simulink model "NPW_Model"  (R2025a)
settings: Solver=VariableStepAuto  StartTime=0.0  StopTime=150.0  RelTol=1e-3
undefined symbols (not defined in the file or in its folder): sim_leak_area, sim_outlet_slope
libraries: fl_lib x58, nesl_utility x5, simulink x3, SimscapeFluids_lib x1
(part 2 of 2)

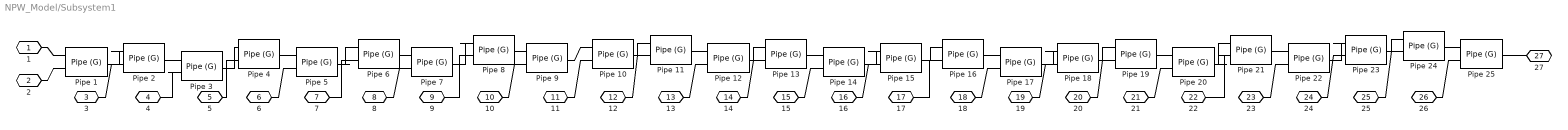
== system NPW_Model/Subsystem1 ==
  Pipe {1..25} (25 alike) : fl_lib/Gas/Elements/Pipe (G)  length=sim_block_L_up m  area=0.19635 m^2  Dh=0.5 m  length_add=0 m  roughness=4.5e-5 m  Re_lam=2000  Re_tur=4000  shape_factor=64  Nu_lam=3.66  dynamic_compressibility=true  inertia=true  p_init=4.5 MPa  p_init_priority=foundation.enum.Priority.None  T_init=293.15 K  T_init_priority=foundation.enum.Priority.None  mdot_init=0 kg/s  mdot_init_priority=foundation.enum.Priority.None  p_nominal=0.101325 MPa  T_nominal=293.15 K
  1 : PMIOPort  Side=Left
  2 : PMIOPort  Port=2  Side=Left
  3 : PMIOPort  Port=3  Side=Left
  4 : PMIOPort  Port=4  Side=Left
  5 : PMIOPort  Port=5  Side=Left
  6 : PMIOPort  Port=6  Side=Left
  7 : PMIOPort  Port=7  Side=Left
  8 : PMIOPort  Port=8  Side=Left
  9 : PMIOPort  Port=9  Side=Left
  10 : PMIOPort  Port=10  Side=Left
  11 : PMIOPort  Port=11  Side=Left
  12 : PMIOPort  Port=12  Side=Left
  13 : PMIOPort  Port=13  Side=Left
  14 : PMIOPort  Port=14  Side=Left
  15 : PMIOPort  Port=15  Side=Left
  16 : PMIOPort  Port=16  Side=Left
  17 : PMIOPort  Port=17  Side=Left
  18 : PMIOPort  Port=18  Side=Left
  19 : PMIOPort  Port=19  Side=Left
  20 : PMIOPort  Port=20  Side=Left
  21 : PMIOPort  Port=21  Side=Left
  22 : PMIOPort  Port=22  Side=Left
  23 : PMIOPort  Port=23  Side=Left
  24 : PMIOPort  Port=24  Side=Left
  25 : PMIOPort  Port=25  Side=Left
  26 : PMIOPort  Port=26  Side=Left
  27 : PMIOPort  Port=27  Side=Right
  connections:
  Pipe 19/LConn2 -- 20/RConn1
  Pipe 13/RConn1 -- Pipe 14/LConn1
  Pipe 17/LConn1 -- Pipe 16/RConn1
  Pipe 13/LConn1 -- Pipe 12/RConn1
  Pipe 10/LConn2 -- 11/RConn1
  Pipe 5/LConn1 -- Pipe 4/RConn1
  Pipe 6/LConn2 -- 7/RConn1
  Pipe 3/LConn2 -- 4/RConn1
  Pipe 10/RConn1 -- Pipe 11/LConn1
  Pipe 15/LConn1 -- Pipe 14/RConn1
  Pipe 12/LConn2 -- 13/RConn1
  Pipe 1/LConn2 -- 2/RConn1
  Pipe 20/RConn1 -- Pipe 21/LConn1
  Pipe 14/LConn2 -- 15/RConn1
  Pipe 15/RConn1 -- Pipe 16/LConn1
  Pipe 12/LConn1 -- Pipe 11/RConn1
  Pipe 22/LConn1 -- Pipe 21/RConn1
  Pipe 2/LConn2 -- 3/RConn1
  Pipe 18/LConn1 -- Pipe 17/RConn1
  Pipe 7/LConn2 -- 8/RConn1
  Pipe 20/LConn1 -- Pipe 19/RConn1
  Pipe 2/LConn1 -- Pipe 1/RConn1
  Pipe 25/RConn1 -- 27/RConn1
  Pipe 20/LConn2 -- 21/RConn1
  Pipe 8/RConn1 -- Pipe 9/LConn1
  Pipe 23/LConn2 -- 24/RConn1
  Pipe 3/LConn1 -- Pipe 2/RConn1
  Pipe 23/LConn1 -- Pipe 22/RConn1
  Pipe 8/LConn1 -- Pipe 7/RConn1
  Pipe 22/LConn2 -- 23/RConn1
  Pipe 10/LConn1 -- Pipe 9/RConn1
  Pipe 7/LConn1 -- Pipe 6/RConn1
  Pipe 11/LConn2 -- 12/RConn1
  Pipe 25/LConn1 -- Pipe 24/RConn1
  Pipe 23/RConn1 -- Pipe 24/LConn1
  Pipe 8/LConn2 -- 9/RConn1
  Pipe 5/RConn1 -- Pipe 6/LConn1
  Pipe 3/RConn1 -- Pipe 4/LConn1
  Pipe 17/LConn2 -- 18/RConn1
  Pipe 18/RConn1 -- Pipe 19/LConn1
  Pipe 9/LConn2 -- 10/RConn1
  Pipe 21/LConn2 -- 22/RConn1
  Pipe 13/LConn2 -- 14/RConn1
  Pipe 24/LConn2 -- 25/RConn1
  Pipe 18/LConn2 -- 19/RConn1
  Pipe 4/LConn2 -- 5/RConn1
  Pipe 5/LConn2 -- 6/RConn1
  Pipe 16/LConn2 -- 17/RConn1
  Pipe 15/LConn2 -- 16/RConn1
  Pipe 1/LConn1 -- 1/RConn1
  Pipe 25/LConn2 -- 26/RConn1

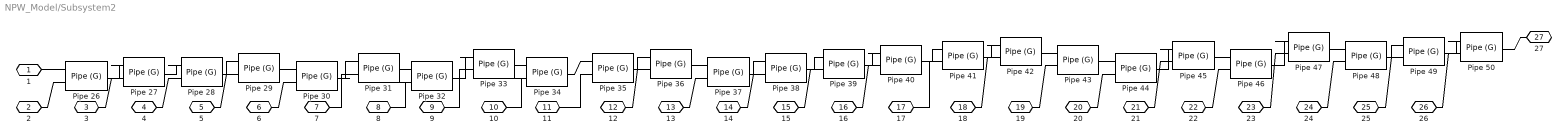
== system NPW_Model/Subsystem2 ==
  Pipe {26..50} (25 alike) : fl_lib/Gas/Elements/Pipe (G)  length=sim_block_L_down m  area=0.19635 m^2  Dh=0.5 m  length_add=0 m  roughness=4.5e-5 m  Re_lam=2000  Re_tur=4000  shape_factor=64  Nu_lam=3.66  dynamic_compressibility=true  inertia=true  p_init=4.5 MPa  p_init_priority=foundation.enum.Priority.None  T_init=293.15 K  T_init_priority=foundation.enum.Priority.None  mdot_init=0 kg/s  mdot_init_priority=foundation.enum.Priority.None  p_nominal=0.101325 MPa  T_nominal=293.15 K
  1 : PMIOPort  Side=Right
  2 : PMIOPort  Port=2  Side=Right
  3 : PMIOPort  Port=3  Side=Right
  4 : PMIOPort  Port=4  Side=Right
  5 : PMIOPort  Port=5  Side=Right
  6 : PMIOPort  Port=6  Side=Right
  7 : PMIOPort  Port=7  Side=Right
  8 : PMIOPort  Port=8  Side=Right
  9 : PMIOPort  Port=9  Side=Right
  10 : PMIOPort  Port=10  Side=Right
  11 : PMIOPort  Port=11  Side=Right
  12 : PMIOPort  Port=12  Side=Right
  13 : PMIOPort  Port=13  Side=Right
  14 : PMIOPort  Port=14  Side=Right
  15 : PMIOPort  Port=15  Side=Right
  16 : PMIOPort  Port=16  Side=Right
  17 : PMIOPort  Port=17  Side=Right
  18 : PMIOPort  Port=18  Side=Right
  19 : PMIOPort  Port=19  Side=Right
  20 : PMIOPort  Port=20  Side=Right
  21 : PMIOPort  Port=21  Side=Right
  22 : PMIOPort  Port=22  Side=Right
  23 : PMIOPort  Port=23  Side=Right
  24 : PMIOPort  Port=24  Side=Right
  25 : PMIOPort  Port=25  Side=Right
  26 : PMIOPort  Port=26  Side=Right
  27 : PMIOPort  Port=27  Side=Left
  connections:
  Pipe 28/LConn1 -- Pipe 27/RConn1
  Pipe 38/LConn1 -- Pipe 37/RConn1
  Pipe 38/LConn2 -- 14/RConn1
  Pipe 49/LConn2 -- 25/RConn1
  Pipe 30/RConn1 -- Pipe 31/LConn1
  Pipe 29/LConn2 -- 5/RConn1
  Pipe 43/LConn2 -- 19/RConn1
  Pipe 28/LConn2 -- 4/RConn1
  Pipe 48/LConn1 -- Pipe 47/RConn1
  Pipe 48/LConn2 -- 24/RConn1
  Pipe 30/LConn2 -- 6/RConn1
  Pipe 48/RConn1 -- Pipe 49/LConn1
  Pipe 30/LConn1 -- Pipe 29/RConn1
  Pipe 36/LConn2 -- 12/RConn1
  Pipe 50/LConn1 -- Pipe 49/RConn1
  Pipe 33/LConn1 -- Pipe 32/RConn1
  Pipe 47/LConn2 -- 23/RConn1
  Pipe 35/LConn1 -- Pipe 34/RConn1
  Pipe 42/LConn1 -- Pipe 41/RConn1
  Pipe 44/LConn2 -- 20/RConn1
  Pipe 40/LConn1 -- Pipe 39/RConn1
  Pipe 33/RConn1 -- Pipe 34/LConn1
  Pipe 33/LConn2 -- 9/RConn1
  Pipe 50/LConn2 -- 26/RConn1
  Pipe 35/LConn2 -- 11/RConn1
  Pipe 43/RConn1 -- Pipe 44/LConn1
  Pipe 27/LConn1 -- Pipe 26/RConn1
  Pipe 47/LConn1 -- Pipe 46/RConn1
  Pipe 37/LConn1 -- Pipe 36/RConn1
  Pipe 35/RConn1 -- Pipe 36/LConn1
  Pipe 31/LConn2 -- 7/RConn1
  Pipe 50/RConn1 -- 27/RConn1
  Pipe 34/LConn2 -- 10/RConn1
  Pipe 28/RConn1 -- Pipe 29/LConn1
  Pipe 38/RConn1 -- Pipe 39/LConn1
  Pipe 32/LConn1 -- Pipe 31/RConn1
  Pipe 45/LConn1 -- Pipe 44/RConn1
  Pipe 40/RConn1 -- Pipe 41/LConn1
  Pipe 43/LConn1 -- Pipe 42/RConn1
  Pipe 26/LConn2 -- 2/RConn1
  Pipe 42/LConn2 -- 18/RConn1
  Pipe 39/LConn2 -- 15/RConn1
  Pipe 45/RConn1 -- Pipe 46/LConn1
  Pipe 32/LConn2 -- 8/RConn1
  Pipe 40/LConn2 -- 16/RConn1
  Pipe 45/LConn2 -- 21/RConn1
  Pipe 26/LConn1 -- 1/RConn1
  Pipe 27/LConn2 -- 3/RConn1
  Pipe 41/LConn2 -- 17/RConn1
  Pipe 46/LConn2 -- 22/RConn1
  Pipe 37/LConn2 -- 13/RConn1
